simulink model "Calculator"  (R2018a)
settings: Solver=FixedStepDiscrete  StartTime=0.0  StopTime=10.0  RelTol=1e-3
settings Model: Creator=Moataz  LastModifiedBy=Moataz
settings OptimizationCC: DefaultParameterBehavior=Inlined  EnhancedBackFolding=on  PassReuseOutputArgsAs=Individual arguments  OptimizeBlockOrder=speed  DifferentSizesBufferReuse=on  OptimizationCustomize=off
settings DebuggingCC: ParameterTunabilityLossMsg=error
settings SFSimCC: MATLABDynamicMemAlloc=off
settings RTWCC: SystemTargetFile=ert.tlc  GenCodeOnly=on  TemplateMakefile=ert_default_tmf  GenerateReport=on  IncludeHyperlinkInReport=on  LaunchReport=on  GenerateTraceInfo=on  GenerateTraceReport=on  GenerateTraceReportSl=on  GenerateTraceReportSf=on  GenerateTraceReportEml=on
settings CodeAppCC: ForceParamTrailComments=on  IgnoreCustomStorageClasses=off  OperatorAnnotations=on  SimulinkDataObjDesc=on  SFDataObjDesc=on  InsertBlockDesc=on
settings ERTTargetCC: TargetLangStandard=C99 (ISO)  GenerateSampleERTMain=on  InlinedParameterPlacement=NonHierarchical  ERTCustomFileTemplate=example_file_process.tlc

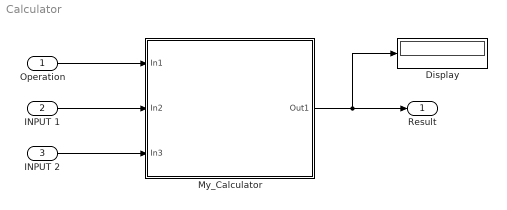
== system Calculator ==
  "Operation " : Inport
  "INPUT 1 " : Inport  Port=2  OutDataTypeStr=int32
  INPUT 2 : Inport  Port=3  OutDataTypeStr=int32
  Display : Display
  My_Calculator : Subsystem  TreatAsAtomicUnit=on
      settings: RTWFcnNameOpts=Use subsystem name  RTWFileNameOpts=Use subsystem name
  "Result " : Outport  OutDataTypeStr=int32
  wires:
  My_Calculator/1(Out1) -> Display/1, "Result "/1
  "Operation "/1 -> My_Calculator/1(In1)
  "INPUT 1 "/1 -> My_Calculator/2(In2)
  INPUT 2/1 -> My_Calculator/3(In3)

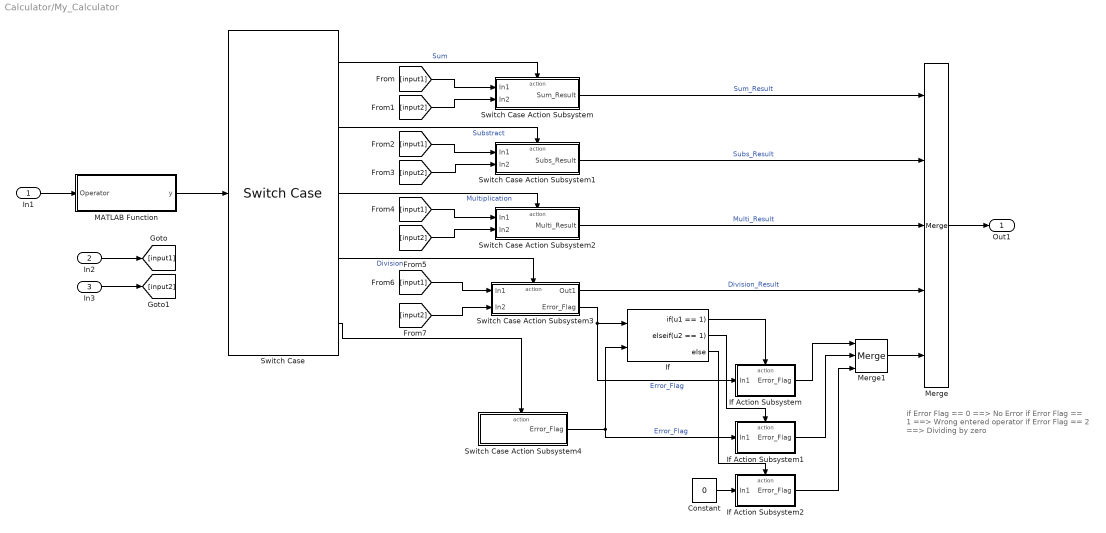
== system Calculator/My_Calculator ==
  note: if Error Flag == 0 ==> No Error
      | if Error Flag == 1 ==> Wrong entered operator
      | if Error Flag == 2 ==> Dividing by zero
  In1 : Inport
  In2 : Inport  Port=2  OutDataTypeStr=int32
  In3 : Inport  Port=3  OutDataTypeStr=int32
  Constant : Constant  Value=0  OutDataTypeStr=int32
  If : If  NumInputs=2  IfExpression=u1 == 1  ElseIfExpressions=u2 == 1
  If Action Subsystem : Subsystem  TreatAsAtomicUnit=on
  If Action Subsystem1 : Subsystem  TreatAsAtomicUnit=on
  If Action Subsystem2 : Subsystem  TreatAsAtomicUnit=on
  MATLAB Function : MATLAB Function  TreatAsAtomicUnit=on
  Merge : Merge  Inputs=5
  Merge1 : Merge  Inputs=3
  Switch Case : SwitchCase  CaseConditions={0 1 2 3}
  Switch Case Action Subsystem : Subsystem  TreatAsAtomicUnit=on
  Switch Case Action Subsystem1 : Subsystem  TreatAsAtomicUnit=on
  Switch Case Action Subsystem2 : Subsystem  TreatAsAtomicUnit=on
  Switch Case Action Subsystem3 : Subsystem  TreatAsAtomicUnit=on
  Switch Case Action Subsystem4 : Subsystem  TreatAsAtomicUnit=on
  Out1 : Outport
  wires:
  Switch Case/1 -> Switch Case Action Subsystem/Action  "Sum"
  MATLAB Function/1(y) -> Switch Case/1
  Switch Case Action Subsystem1/1(Subs_Result) -> Merge/2  "Subs_Result"
  Switch Case/4 -> Switch Case Action Subsystem3/Action  "Division"
  [input1] -> Switch Case Action Subsystem3/1(In1)
  Switch Case Action Subsystem2/1(Multi_Result) -> Merge/3  "Multi_Result"
  [input2] -> Switch Case Action Subsystem3/2(In2)
  Switch Case/2 -> Switch Case Action Subsystem1/Action  "Substract"
  Merge/1 -> Out1/1
  [input1] -> Switch Case Action Subsystem/1(In1)
  [input2] -> Switch Case Action Subsystem1/2(In2)
  [input1] -> Switch Case Action Subsystem1/1(In1)
  Switch Case Action Subsystem/1(Sum_Result) -> Merge/1  "Sum_Result"
  Switch Case/3 -> Switch Case Action Subsystem2/Action  "Multiplication"
  [input1] -> Switch Case Action Subsystem2/1(In1)
  [input2] -> Switch Case Action Subsystem2/2(In2)
  In1/1 -> MATLAB Function/1(Operator)
  [input2] -> Switch Case Action Subsystem/2(In2)
  In3/1 -> [input2]
  In2/1 -> [input1]
  Switch Case/5 -> Switch Case Action Subsystem4/Action
  If/2 -> If Action Subsystem1/Action
  If/1 -> If Action Subsystem/Action
  Switch Case Action Subsystem3/1(Out1) -> Merge/4  "Division_Result"
  If Action Subsystem/1(Error_Flag) -> Merge1/1
  If Action Subsystem1/1(Error_Flag) -> Merge1/2
  If Action Subsystem2/1(Error_Flag) -> Merge1/3
  Merge1/1 -> Merge/5
  If/3 -> If Action Subsystem2/Action
  Constant/1 -> If Action Subsystem2/1(In1)
  Switch Case Action Subsystem4/1(Error_Flag) -> If Action Subsystem1/1(In1), If/2  "Error_Flag"
  Switch Case Action Subsystem3/2(Error_Flag) -> If/1, If Action Subsystem/1(In1)  "Error_Flag"

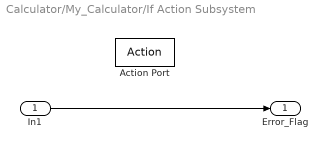
== system Calculator/My_Calculator/If Action Subsystem ==
  In1 : Inport  OutDataTypeStr=int32
  Action Port : ActionPort  ActionType=then
  Error_Flag : Outport  OutDataTypeStr=int32
  wires:
  In1/1 -> Error_Flag/1

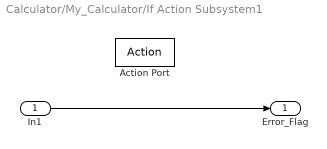
== system Calculator/My_Calculator/If Action Subsystem1 ==
  In1 : Inport
  Action Port : ActionPort  ActionType=elseif
  Error_Flag : Outport
  wires:
  In1/1 -> Error_Flag/1

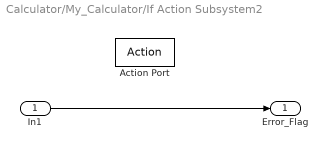
== system Calculator/My_Calculator/If Action Subsystem2 ==
  In1 : Inport
  Action Port : ActionPort  ActionType=else
  Error_Flag : Outport
  wires:
  In1/1 -> Error_Flag/1

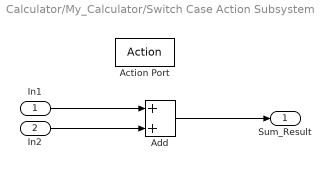
== system Calculator/My_Calculator/Switch Case Action Subsystem ==
  In1 : Inport
  In2 : Inport  Port=2
  Action Port : ActionPort  ActionType=case
  Add : Sum
  Sum_Result : Outport
  wires:
  In2/1 -> Add/2
  In1/1 -> Add/1
  Add/1 -> Sum_Result/1

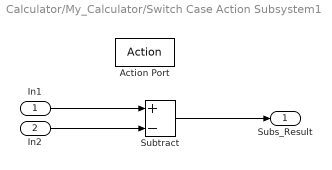
== system Calculator/My_Calculator/Switch Case Action Subsystem1 ==
  In1 : Inport
  In2 : Inport  Port=2
  Action Port : ActionPort  ActionType=case
  Subtract : Sum  Inputs=+-
  Subs_Result : Outport
  wires:
  Subtract/1 -> Subs_Result/1
  In1/1 -> Subtract/1
  In2/1 -> Subtract/2

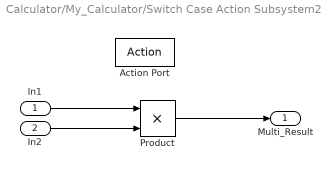
== system Calculator/My_Calculator/Switch Case Action Subsystem2 ==
  In1 : Inport
  In2 : Inport  Port=2
  Action Port : ActionPort  ActionType=case
  Product : Product  OutDataTypeStr=int32
  Multi_Result : Outport  OutDataTypeStr=int32
  wires:
  In2/1 -> Product/2
  In1/1 -> Product/1
  Product/1 -> Multi_Result/1

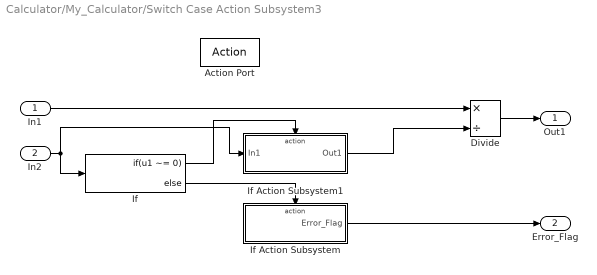
== system Calculator/My_Calculator/Switch Case Action Subsystem3 ==
  In1 : Inport
  In2 : Inport  Port=2
  Action Port : ActionPort  ActionType=case
  Divide : Product  Inputs=*/
  If : If  IfExpression=u1 ~= 0
  If Action Subsystem : Subsystem  TreatAsAtomicUnit=on
  If Action Subsystem1 : Subsystem  TreatAsAtomicUnit=on
  Out1 : Outport  OutDataTypeStr=int32
  Error_Flag : Outport  Port=2  OutDataTypeStr=int32
  wires:
  In1/1 -> Divide/1
  In2/1 -> If Action Subsystem1/1(In1), If/1
  If/2 -> If Action Subsystem/Action
  If/1 -> If Action Subsystem1/Action
  Divide/1 -> Out1/1
  If Action Subsystem1/1(Out1) -> Divide/2
  If Action Subsystem/1(Error_Flag) -> Error_Flag/1

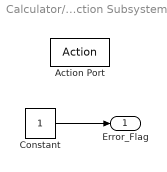
== system Calculator/My_Calculator/Switch Case Action Subsystem4 ==
  Action Port : ActionPort  ActionType=default
  Constant : Constant  OutDataTypeStr=int32
  Error_Flag : Outport  OutDataTypeStr=int32
  wires:
  Constant/1 -> Error_Flag/1

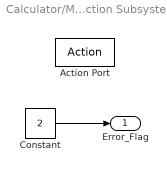
== system Calculator/My_Calculator/Switch Case Action Subsystem3/If Action Subsystem ==
  Action Port : ActionPort  ActionType=else
  Constant : Constant  Value=2  OutDataTypeStr=int32
  Error_Flag : Outport  OutDataTypeStr=int32
  wires:
  Constant/1 -> Error_Flag/1

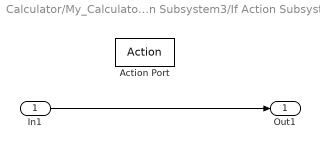
== system Calculator/My_Calculator/Switch Case Action Subsystem3/If Action Subsystem1 ==
  In1 : Inport
  Action Port : ActionPort  ActionType=then
  Out1 : Outport
  wires:
  In1/1 -> Out1/1

== matlab function Calculator/My_Calculator/MATLAB Function ==
  data: Operator input; y output
function y = fcn(Operator)
y=0;
switch Operator
    case '+'
        y=0;
    case '-'
        y=1;
    case '*'
        y=2;
    case '/'
        y=3;
    otherwise
        y=4;
end
